simulink library "Px4Library"  (R2015b)
settings: Solver=VariableStepAuto  StartTime=0.0  StopTime=10.0  RelTol=1e-3
undefined symbols (not defined in the file): armed, ctrl_state, INIT_PARAM_VECTOR, mpc_att_sp, mpc_ctrl_state, mpc_manual, mpc_pos_sp_triplet, mpc_vehicle_land_detected, mpc_vehicle_status, v_att_sp, v_control_mode
libraries: simulink x4
(part 6 of 7)

== matlab function Px4Library/Quadcopter mixer/mixer ==
  data: inputControl input; outputControl output
function outputControl = mix( inputControl )
%#codegen
% MIX mix control input
%     inputControl(1) = inputControl(1);
%     inputControl(2) = inputControl(2);
%     inputControl(3) = inputControl(3);
    
    ROTOR_COUNT = 4;
    rotors = struct('roll_scale',  {-0.707107,  0.707107, 0.707107, -0.707107}, ...
                    'pitch_scale', { 0.707107, -0.707107, 0.707107, -0.707107}, ...
                    'yaw_scale',   { 1.00,      1.00,    -1.00,     -1.00});

    roll   = constrain(inputControl(1), -1.0, 1.0);
    pitch  = constrain(inputControl(2), -1.0, 1.0);
    yaw    = constrain(inputControl(3), -1.0, 1.0);
    thrust = constrain(inputControl(4), 0.0, 1.0);
    min_out = 0.0;
    max_out = 0.0;
    
    outputControl = zeros(ROTOR_COUNT,1);

    % /* perform initial mix pass yielding unbounded outputs, ignore yaw */
    for i = 1:ROTOR_COUNT % ROTOR COUNT!!! %(unsigned i = 0; i < _rotor_count; i++)
         out = roll * rotors(i).roll_scale ...
                + pitch * rotors(i).pitch_scale + thrust;

        % /* limit yaw if it causes outputs clipping */
        if ( (out >= 0.0) && (out < (-yaw * rotors(i).yaw_scale) ) )
            yaw = -out / rotors(i).yaw_scale;
        end

        % /* calculate min and max output values */
        if (out < min_out)
            min_out = out;
        end

        if (out > max_out)
            max_out = out;
        end

        outputControl(i) = out;
    end

    % /* scale down roll/pitch controls if some outputs are negative, don't add yaw, keep total thrust */
    if (min_out < 0.0)
         scale_in = thrust / (thrust - min_out);

        % /* mix again with adjusted controls */
        for i = 1:ROTOR_COUNT %(unsigned i = 0; i < _rotor_count; i++)
            outputControl(i) = scale_in ...
                         * (roll * rotors(i).roll_scale ...
                        + pitch * rotors(i).pitch_scale) + thrust;
        end
    else
        % /* roll/pitch mixed without limiting, add yaw control */
        for i=1:ROTOR_COUNT %(unsigned i = 0; i < _rotor_count; i++)
            outputControl(i) = outputControl(i) + yaw * rotors(i).yaw_scale;
        end
    end

    % /* scale down all outputs if some outputs are too large, reduce total thrust */
    % scale_out;

    if (max_out > 1.0)
        scale_out = 1.0 / max_out;

    else
        scale_out = 1.0;
    end

    % /* scale outputs to range _idle_speed..1, and do final limiting */
    for i=1:ROTOR_COUNT %(unsigned i = 0; i < _rotor_count; i++)
        outputControl(i) = constrain(outputControl(i) * scale_out, 0.0, 1.0); % added scale_out
    end

end

function y = constrain( x, x_min, x_max )
    y = max( min(x, x_max), x_min );
end

== matlab function Px4Library/local_position_estimator/Output selection ==
  data: est_status_covariances output; est_status_health_flags output; est_status_states output; gpos_vel_n output; gpos_vel_e output; selfVec input; gpos_vel_d output; lpos_vx output; lpos_vy output; lpos_vz output; lpos_x output; lpos_y output; lpos_z output; lpos_yaw output
function [ ...
                   est_status_covariances, ...
                  est_status_health_flags, ...
                        est_status_states, ...
                               gpos_vel_n, ...
                               gpos_vel_e, ...
                               gpos_vel_d, ...
                                  lpos_vx, ...
                                  lpos_vy, ...
                                  lpos_vz, ...
                                   lpos_x, ...
                                   lpos_y, ...
                                   lpos_z, ...
                                 lpos_yaw] ...
   = OutputSelection( selfVec )
%#codegen

	% Variable assignment
	                  est_status_covariances = selfVec(439:448);
	                 est_status_health_flags = selfVec(449:449);
	                       est_status_states = selfVec(454:463);
	                              gpos_vel_n = selfVec(480:480);
	                              gpos_vel_e = selfVec(481:481);
	                              gpos_vel_d = selfVec(482:482);
	                                 lpos_vx = selfVec(501:501);
	                                 lpos_vy = selfVec(502:502);
	                                 lpos_vz = selfVec(503:503);
	                                  lpos_x = selfVec(504:504);
	                                  lpos_y = selfVec(507:507);
	                                  lpos_z = selfVec(508:508);
	                                lpos_yaw = selfVec(512:512);
end

== matlab function Px4Library/PX4 rotor map to sim rotor map/PX4 motor map to sim motor map ==
  data: px4Pwm input; simPwm output
function simPwm = motor_map(px4Pwm)
%#codegen

simPwm = [ px4Pwm(3); px4Pwm(2); px4Pwm(4); px4Pwm(1) ];

== matlab function Px4Library/attitude_estimator_q/Input assignment q ==
  data: airspeed_sub_indicated_airspeed_m_s input; airspeed_sub_timestamp input; airspeed_sub_updated input; mocap_sub_updated input; mocap_sub_q input; mocap_sub_timestamp input; sensors_sub_updated input; sensors_sub_timestamp input; sensors_sub_gyro_rad input; sensors_sub_accelerometer_m_s2 input; sensors_sub_accelerometer_timestamp_relative input; sensors_sub_magnetometer_ga input; sensors_sub_magnetometer_timestamp_relative input; selfVecIn input; selfVec output
function selfVec = InputAssignment( ...
	     airspeed_sub_indicated_airspeed_m_s, ...
	                  airspeed_sub_timestamp, ...
	                    airspeed_sub_updated, ...
	                       mocap_sub_updated, ...
	                             mocap_sub_q, ...
	                     mocap_sub_timestamp, ...
	                     sensors_sub_updated, ...
	                   sensors_sub_timestamp, ...
	                    sensors_sub_gyro_rad, ...
	          sensors_sub_accelerometer_m_s2, ...
	sensors_sub_accelerometer_timestamp_relative, ...
	             sensors_sub_magnetometer_ga, ...
	sensors_sub_magnetometer_timestamp_relative, ...
	                               selfVecIn ...
	)
%#codegen

	selfVec = selfVecIn;

	% Variable assignment
	selfVec( 9: 9) =      airspeed_sub_indicated_airspeed_m_s;
	selfVec(10:10) =                   airspeed_sub_timestamp;
	selfVec(11:11) =                     airspeed_sub_updated;
	selfVec(135:135) =                        mocap_sub_updated;
	selfVec(136:139) =                              mocap_sub_q;
	selfVec(140:140) =                      mocap_sub_timestamp;
	selfVec(153:153) =                      sensors_sub_updated;
	selfVec(154:154) =                    sensors_sub_timestamp;
	selfVec(155:157) =                     sensors_sub_gyro_rad;
	selfVec(158:160) =           sensors_sub_accelerometer_m_s2;
	selfVec(161:161) = sensors_sub_accelerometer_timestamp_relative;
	selfVec(162:164) =              sensors_sub_magnetometer_ga;
	selfVec(165:165) = sensors_sub_magnetometer_timestamp_relative;
end

== matlab function Px4Library/attitude_estimator_q/Output selection q ==
  data: att_pub_timestamp output; att_pub_rollspeed output; att_pub_pitchspeed output; att_pub_yawspeed output; att_pub_q output; selfVec input
function [ ...
                        att_pub_timestamp, ...
                        att_pub_rollspeed, ...
                       att_pub_pitchspeed, ...
                         att_pub_yawspeed, ...
                                att_pub_q] ...
   = OutputSelection( selfVec )
%#codegen

	% Variable assignment
	                       att_pub_timestamp = selfVec(12:12);
	                       att_pub_rollspeed = selfVec(13:13);
	                      att_pub_pitchspeed = selfVec(14:14);
	                        att_pub_yawspeed = selfVec(15:15);
	                               att_pub_q = selfVec(16:19);
end
